simulink model "Arm_2DOF_Step_Input"  (R2021a)
settings: Solver=VariableStepAuto  StartTime=0.0  StopTime=5  MaxStep=0.01  RelTol=1e-3
settings Model: EnablePacing=on  PacingRate=8  Creator=Zicx  LastModifiedBy=Zicx
settings SolverCC: MaxConsecutiveZCs=1500  MaxConsecutiveMinStep=100  ZeroCrossAlgorithm=Adaptive
settings DebuggingCC: SignalInfNanChecking=error  MaskedZcDiagnostic=none  IgnoredZcDiagnostic=none  CheckMatrixSingularityMsg=error  FixptConstUnderflowMsg=warning  FixptConstOverflowMsg=warning  FixptConstPrecisionLossMsg=warning  VectorMatrixConversionMsg=warning  UnderSpecifiedDimensionMsg=error

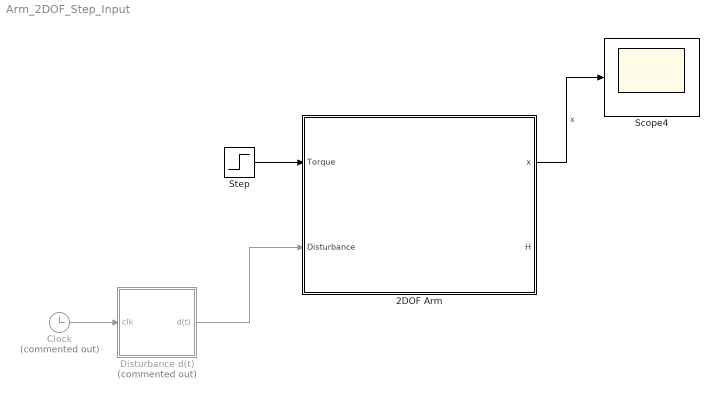
== system Arm_2DOF_Step_Input ==
  2DOF Arm : Subsystem
  Clock : Clock  Commented=on
  Disturbance d(t) : Subsystem  Commented=on
  Scope4 : Scope
  Step : Step  After=[1;1]  SampleTime=0  VectorParams1D=off
  wires:
  Disturbance d(t)/1(d(t)) -> 2DOF Arm/2(Disturbance)
  2DOF Arm/1(x) -> Scope4/1  "x"
  Clock/1 -> Disturbance d(t)/1(clk)
  Step/1 -> 2DOF Arm/1(Torque)

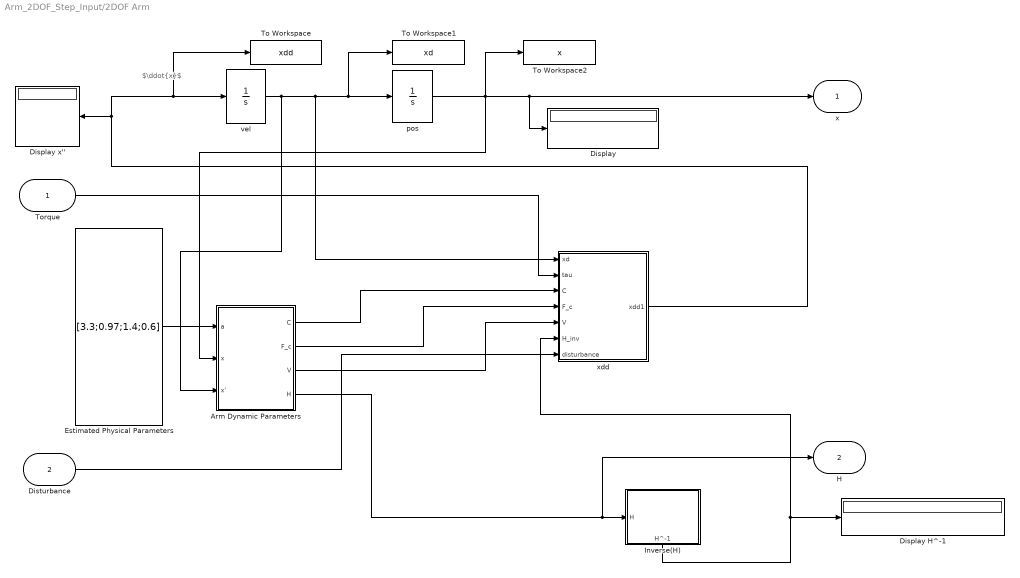
== system Arm_2DOF_Step_Input/2DOF Arm ==
  note: $\ddot{x}$
  Torque : Inport  OutDataTypeStr=double  PortDimensions=[2 1]
  Disturbance : Inport  Port=2  PortDimensions=[2 1]
  Arm Dynamic Parameters : Subsystem
  Display : Display
  Display H^-1 : Display
  Display x'' : Display
  Estimated Physical Parameters : Constant  Value=[3.3;0.97;1.4;0.6]
  Inverse(H) : Subsystem
      settings: PortSchema="{\"entries\":[{\"content\":{\"sides\":[{\"content\":{\"connectorIds\":[\"In1\"]},\"type\":\"ConnectorPlacement.EquallySpacedRectSide\",\"uuid\":\"e93da7b9-99f6-499c-a0cb-6f5b129eec99\"},{\"content\":{\"connectorIds\":[],\"side\":\"RIGHT\"},\"type\":\"ConnectorPlacement.EquallySpacedRectSide\",\"uuid\":\"25c75cce-7d31-4940-9360-78f60f805e3f\"},{\"content\":{\"connectorIds\":[],\"side\":\"TOP\"},\"type\":\"ConnectorPlacement.EquallySpacedRectSide\",\"uuid\":\"446b159b-687d-4bab-aeef-b2e357b1c9d1\"},{\"content\":{\"connectorIds\":[\"Out1\"],\"side\":\"BOTTOM\"},\"type\":\"ConnectorPlacement.EquallySpacedRectSide\",\"uuid\":\"0391da42-abcf-4982-934b-6703b1b91c15\"}]},\"type\":\"ConnectorPlacement.EquallySpacedConnector\",\"uuid\":\"51b5e751-d260-4a7c-9da1-3f7a116869ab\"}],\"packageUris\":[\"http://schema.mathworks.com/mf0/Connector/R2020b\"],\"version\":\"1.0\"}"
  To Workspace : ToWorkspace  VariableName=xdd  SaveFormat=Timeseries  SampleTime=-1
  To Workspace1 : ToWorkspace  VariableName=xd  SaveFormat=Timeseries  SampleTime=-1
  To Workspace2 : ToWorkspace  VariableName=x  SaveFormat=Structure With Time  SampleTime=-1
  pos : Integrator  InitialCondition=[0.3;0.5]  LimitOutput=on  UpperSaturationLimit=2*pi  LowerSaturationLimit=-2 * pi  ContinuousStateAttributes='pos'
  vel : Integrator  LimitOutput=on  UpperSaturationLimit=2*pi  LowerSaturationLimit=-2*pi  ContinuousStateAttributes='vel'
  xdd : Subsystem
  x : Outport  OutDataTypeStr=double  PortDimensions=[2 1]  SampleTime=0
  H : Outport  Port=2
  wires:
  Estimated Physical Parameters/1 -> Arm Dynamic Parameters/1(a)
  Inverse(H)/1(H^-1) -> xdd/6(H_inv), Display H^-1/1
  Arm Dynamic Parameters/4(H) -> H/1, Inverse(H)/1(H)
  vel/1 -> Arm Dynamic Parameters/3(x'), xdd/1(xd), To Workspace1/1, pos/1
  pos/1 -> To Workspace2/1, Arm Dynamic Parameters/2(x), Display/1, x/1
  xdd/1(xdd1) -> Display x''/1, To Workspace/1, vel/1
  Torque/1 -> xdd/2(tau)
  Arm Dynamic Parameters/1(C) -> xdd/3(C)
  Arm Dynamic Parameters/2(F_c) -> xdd/4(F_c)
  Arm Dynamic Parameters/3(V) -> xdd/5(V)
  Disturbance/1 -> xdd/7(disturbance)

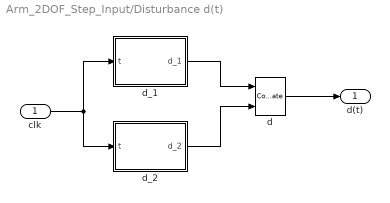
== system Arm_2DOF_Step_Input/Disturbance d(t) ==
  clk : Inport
  d : Concatenate
  d_1 : MATLAB Function  TreatAsAtomicUnit=on
  d_2 : MATLAB Function  TreatAsAtomicUnit=on
  d(t) : Outport
  wires:
  d/1 -> d(t)/1
  clk/1 -> d_2/1(t), d_1/1(t)
  d_1/1(d_1) -> d/1
  d_2/1(d_2) -> d/2

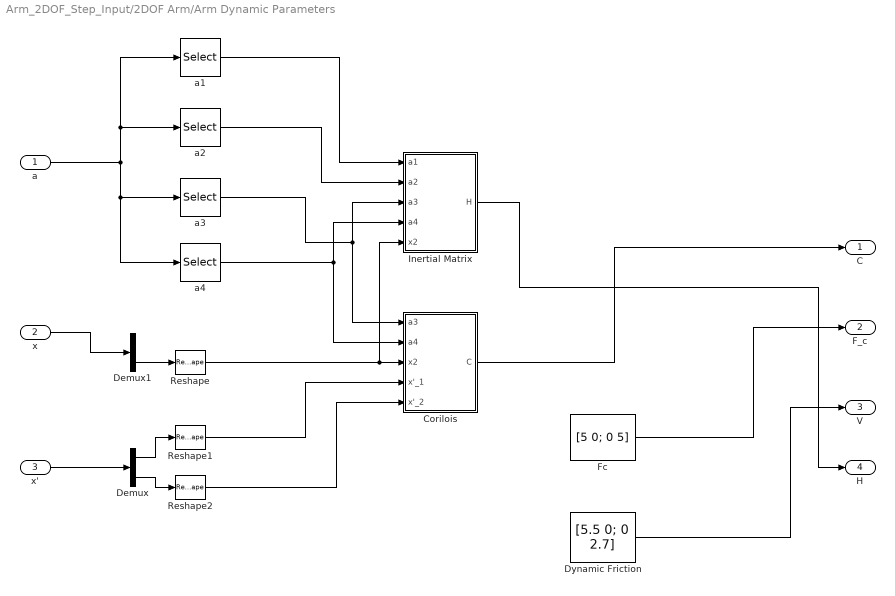
== system Arm_2DOF_Step_Input/2DOF Arm/Arm Dynamic Parameters ==
  a : Inport
  x : Inport  Port=2  PortDimensions=[2 1]
  x' : Inport  Port=3  PortDimensions=[2 1]
  Corilois : Subsystem
  Demux : Demux  Outputs=2
  Demux1 : Demux  Outputs=2
  Dynamic Friction : Constant  Value=[5.5 0; 0 2.7]
  Fc : Constant  Value=[5 0; 0 5]
  Inertial Matrix : Subsystem
  Reshape : Reshape  OutputDimensionality=Customize  OutputDimensions=1
  Reshape1 : Reshape  OutputDimensionality=Customize  OutputDimensions=1
  Reshape2 : Reshape  OutputDimensionality=Customize  OutputDimensions=1
  a1 : Selector  InputPortWidth=4  IndexOptions=Index vector (dialog)  Indices=[1]  OutputSizes=1
  a2 : Selector  InputPortWidth=4  IndexOptions=Index vector (dialog)  Indices=[2]  OutputSizes=1
  a3 : Selector  InputPortWidth=4  IndexOptions=Index vector (dialog)  Indices=[3]  OutputSizes=1
  a4 : Selector  InputPortWidth=4  IndexOptions=Index vector (dialog)  Indices=[4]  OutputSizes=1
  C : Outport
  F_c : Outport  Port=2
  V : Outport  Port=3
  H : Outport  Port=4
  wires:
  a1/1 -> Inertial Matrix/1(a1)
  a/1 -> a1/1, a2/1, a4/1, a3/1
  a3/1 -> Corilois/1(a3), Inertial Matrix/3(a3)
  a4/1 -> Inertial Matrix/4(a4), Corilois/2(a4)
  a2/1 -> Inertial Matrix/2(a2)
  Inertial Matrix/1(H) -> H/1
  Corilois/1(C) -> C/1
  x/1 -> Demux1/1
  Fc/1 -> F_c/1
  Dynamic Friction/1 -> V/1
  x'/1 -> Demux/1
  Demux1/2 -> Reshape/1
  Reshape/1 -> Inertial Matrix/5(x2), Corilois/3(x2)
  Demux/1 -> Reshape1/1
  Demux/2 -> Reshape2/1
  Reshape1/1 -> Corilois/4(x'_1)
  Reshape2/1 -> Corilois/5(x'_2)

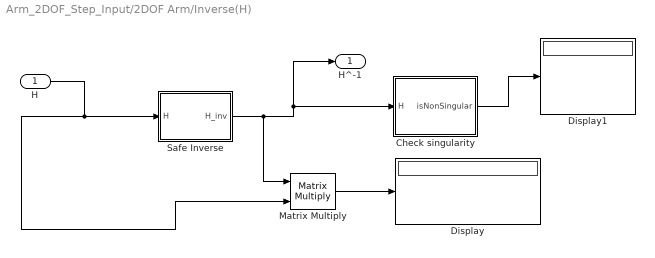
== system Arm_2DOF_Step_Input/2DOF Arm/Inverse(H) ==
  H : Inport  PortDimensions=[2 2]
  Check singularity : MATLAB Function  TreatAsAtomicUnit=on
  Display : Display
  Display1 : Display
  Matrix Multiply : Product  Multiplication=Matrix(*)
  Safe Inverse : MATLAB Function  TreatAsAtomicUnit=on
  H^-1 : Outport
  wires:
  Safe Inverse/1(H_inv) -> Matrix Multiply/1, H^-1/1, Check singularity/1(H)
  H/1 -> Safe Inverse/1(H), Matrix Multiply/2
  Matrix Multiply/1 -> Display/1
  Check singularity/1(isNonSingular) -> Display1/1

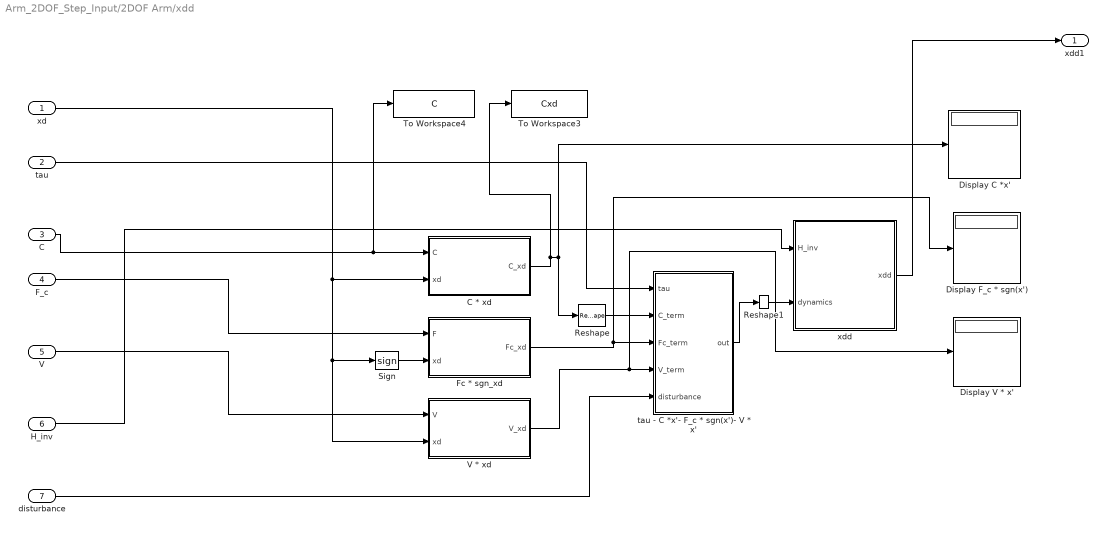
== system Arm_2DOF_Step_Input/2DOF Arm/xdd ==
  xd : Inport
  tau : Inport  Port=2
  C : Inport  Port=3
  F_c : Inport  Port=4
  V : Inport  Port=5
  H_inv : Inport  Port=6
  disturbance : Inport  Port=7
  "C * xd " : MATLAB Function  TreatAsAtomicUnit=on
  Display C *x' : Display
  Display F_c * sgn(x') : Display
  Display V * x' : Display
  Fc * sgn_xd : MATLAB Function  TreatAsAtomicUnit=on
  Reshape : Reshape  OutputDimensionality=Column vector (2-D)
  Reshape1 : Reshape  OutputDimensionality=Column vector (2-D)
  Sign : Signum
  To Workspace3 : ToWorkspace  VariableName=Cxd  SaveFormat=Structure With Time  SampleTime=-1
  To Workspace4 : ToWorkspace  VariableName=C  SaveFormat=Timeseries  SampleTime=-1
  V * xd : MATLAB Function  TreatAsAtomicUnit=on
  "tau - C *x'- F_c * sgn(x')- V * x'  " : MATLAB Function  TreatAsAtomicUnit=on
  xdd : MATLAB Function  TreatAsAtomicUnit=on
  xdd1 : Outport
  wires:
  Sign/1 -> Fc * sgn_xd/2(xd)
  "tau - C *x'- F_c * sgn(x')- V * x'  "/1(out) -> Reshape1/1
  Fc * sgn_xd/1(Fc_xd) -> Display F_c * sgn(x')/1, "tau - C *x'- F_c * sgn(x')- V * x'  "/3(Fc_term)
  xd/1 -> V * xd/2(xd), Sign/1, "C * xd "/2(xd)
  V * xd/1(V_xd) -> Display V * x'/1, "tau - C *x'- F_c * sgn(x')- V * x'  "/4(V_term)
  H_inv/1 -> xdd/1(H_inv)
  Reshape/1 -> "tau - C *x'- F_c * sgn(x')- V * x'  "/2(C_term)
  "C * xd "/1(C_xd) -> To Workspace3/1, Reshape/1, Display C *x'/1
  C/1 -> To Workspace4/1, "C * xd "/1(C)
  Reshape1/1 -> xdd/2(dynamics)
  tau/1 -> "tau - C *x'- F_c * sgn(x')- V * x'  "/1(tau)
  xdd/1(xdd) -> xdd1/1
  disturbance/1 -> "tau - C *x'- F_c * sgn(x')- V * x'  "/5(disturbance)
  V/1 -> V * xd/1(V)
  F_c/1 -> Fc * sgn_xd/1(F)

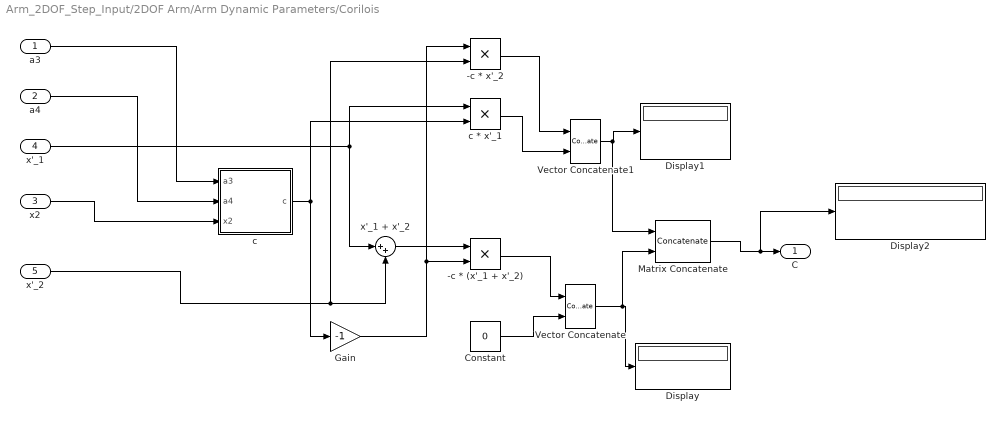
== system Arm_2DOF_Step_Input/2DOF Arm/Arm Dynamic Parameters/Corilois ==
  a3 : Inport
  a4 : Inport  Port=2
  x2 : Inport  Port=3
  x'_1 : Inport  Port=4
  x'_2 : Inport  Port=5
  -c * (x'_1 + x'_2) : Product
  -c * x'_2 : Product
  Constant : Constant  Value=0
  Display : Display
  Display1 : Display
  Display2 : Display
  Gain : Gain  Gain=-1
  Matrix Concatenate : Concatenate  Mode=Multidimensional array  ConcatenateDimension=2
  Vector Concatenate : Concatenate
  Vector Concatenate1 : Concatenate
  c : Subsystem
  c * x'_1 : Product
  x'_1 + x'_2 : Sum  Inputs=|++
  C : Outport
  wires:
  Matrix Concatenate/1 -> Display2/1, C/1
  a4/1 -> c/2(a4)
  a3/1 -> c/1(a3)
  Vector Concatenate1/1 -> Matrix Concatenate/1, Display1/1
  x'_1/1 -> x'_1 + x'_2/1, c * x'_1/1
  x2/1 -> c/3(x2)
  c/1(c) -> Gain/1, c * x'_1/2
  x'_2/1 -> x'_1 + x'_2/2, -c * x'_2/2
  x'_1 + x'_2/1 -> -c * (x'_1 + x'_2)/1
  Vector Concatenate/1 -> Matrix Concatenate/2, Display/1
  Gain/1 -> -c * x'_2/1, -c * (x'_1 + x'_2)/2
  -c * x'_2/1 -> Vector Concatenate1/1
  c * x'_1/1 -> Vector Concatenate1/2
  -c * (x'_1 + x'_2)/1 -> Vector Concatenate/1
  Constant/1 -> Vector Concatenate/2

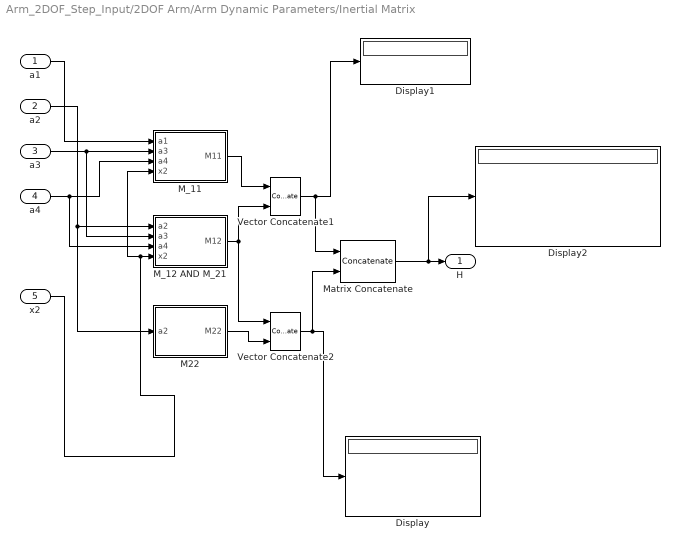
== system Arm_2DOF_Step_Input/2DOF Arm/Arm Dynamic Parameters/Inertial Matrix ==
  a1 : Inport
  a2 : Inport  Port=2
  a3 : Inport  Port=3
  a4 : Inport  Port=4
  x2 : Inport  Port=5
  Display : Display
  Display1 : Display
  Display2 : Display
  M22 : MATLAB Function  TreatAsAtomicUnit=on
  M_11 : MATLAB Function  TreatAsAtomicUnit=on
  M_12 AND M_21 : MATLAB Function  TreatAsAtomicUnit=on
  Matrix Concatenate : Concatenate  Mode=Multidimensional array  ConcatenateDimension=2
  Vector Concatenate1 : Concatenate
  Vector Concatenate2 : Concatenate
  H : Outport
  wires:
  Matrix Concatenate/1 -> Display2/1, H/1
  a1/1 -> M_11/1(a1)
  a3/1 -> M_11/2(a3), M_12 AND M_21/2(a3)
  a4/1 -> M_11/3(a4), M_12 AND M_21/3(a4)
  a2/1 -> M22/1(a2), M_12 AND M_21/1(a2)
  Vector Concatenate2/1 -> Display/1, Matrix Concatenate/2
  M22/1(M22) -> Vector Concatenate2/2
  Vector Concatenate1/1 -> Display1/1, Matrix Concatenate/1
  M_12 AND M_21/1(M12) -> Vector Concatenate2/1, Vector Concatenate1/2
  M_11/1(M11) -> Vector Concatenate1/1
  x2/1 -> M_11/4(x2), M_12 AND M_21/4(x2)

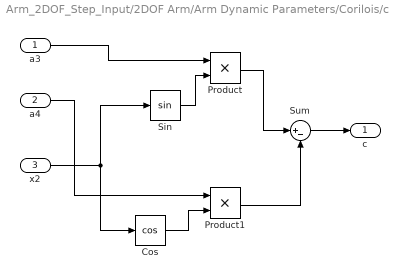
== system Arm_2DOF_Step_Input/2DOF Arm/Arm Dynamic Parameters/Corilois/c ==
  a3 : Inport
  a4 : Inport  Port=2
  x2 : Inport  Port=3
  Cos : Trigonometry  Operator=cos
  Product : Product
  Product1 : Product
  Sin : Trigonometry
  Sum : Sum  Inputs=|+-
  c : Outport
  wires:
  a3/1 -> Product/1
  x2/1 -> Cos/1, Sin/1
  Sin/1 -> Product/2
  a4/1 -> Product1/1
  Cos/1 -> Product1/2
  Product/1 -> Sum/1
  Product1/1 -> Sum/2
  Sum/1 -> c/1

== matlab function Arm_2DOF_Step_Input/2DOF Arm/Inverse(H)/Safe Inverse ==
  data: H input; H_inv output
function H_inv = safe_inverse(H)
    cond_num = cond(H);
    if cond_num > 1e12
        disp('Warning: Matrix is close to singular or badly scaled. Consider using pinv instead.');
        H_inv = pinv(H);
    else
        % Use regularized inverse if necessary
        epsilon = 1e-6; % Small regularization term
        H_reg = H + epsilon * eye(size(H));
        H_inv = inv(H_reg);
        if any(isnan(H_inv), 'all') || any(isinf(H_inv), 'all')
            disp('Warning: Matrix inversion failed. Using pseudoinverse');
            H_inv = pinv(H);
        end
    end
end

== matlab function Arm_2DOF_Step_Input/2DOF Arm/xdd/C * xd  ==
  data: C input; C_xd output; xd input
function C_xd = regulateC_term(C, xd)

    % Define replacement values
    nan_replacement = eps; % A very small positive number
    inf_replacement = realmax; % The largest positive floating-point number
    %negative_inf_replacement = realmin;
    
    % Compute the initial multiplication
    initial_result = C *xd;
    reshape(initial_result, 2, 1);
    
    % Check for NaNs or Infs in the result
    if any(isnan(initial_result)) || any(isinf(initial_result))
        disp("NaN detected in C term!");
    
        % Handle NaNs and Infs in C
        C(isnan(C)) = nan_replacement; % Set NaN elements in C to 0
        C(isinf(C)) = inf_replacement; % Set inf elements in C to 0

        % Handle NaNs and Infs in x_dot
        xd(isnan(xd)) = nan_replacement; % Set NaN elements in x_dot to 0
        xd(isinf(xd)) = inf_replacement; % Set inf elements in x_dot to 0

        % Recompute the multiplication after handling NaNs and Infs
        result = initial_result;
        
        % Ensure the output does not contain NaNs or Infs
        result(isnan(result)) = nan_replacement;
        result(isinf(result)) = inf_replacement;
    else
        % If there are no NaNs or Infs, use the initial result
        result = initial_result;
    end
C_xd = result;
end

== matlab function Arm_2DOF_Step_Input/Disturbance d(t)/d_1 ==
  data: t input; d_1 output
function d_1 = fcn(t)

d_1 = 300* cos(1.7*pi*(t+12)) + 270* sin(pi*t);

== matlab function Arm_2DOF_Step_Input/Disturbance d(t)/d_2 ==
  data: t input; d_2 output
function d_2 = fcn(t)

d_2 = 250 * sin(1.35*pi*(t + 12)) + 300 * cos(2*t);

== matlab function Arm_2DOF_Step_Input/2DOF Arm/Arm Dynamic Parameters/Inertial Matrix/M22 ==
  data: a2 input; M22 output
function M22 = fcn(a2)

M22 = a2;

== matlab function Arm_2DOF_Step_Input/2DOF Arm/Arm Dynamic Parameters/Inertial Matrix/M_11 ==
  data: a1 input; a3 input; a4 input; M11 output; x2 input
function M11 = fcn(a1, a3, a4, x2)
%#codegen

M11 = a1 + 2*a3 * cos(x2)- 2 * a4 * sin(x2);

== matlab function Arm_2DOF_Step_Input/2DOF Arm/Arm Dynamic Parameters/Inertial Matrix/M_12 AND M_21 ==
  data: a2 input; M12 output; a3 input; a4 input; x2 input
function M12 = fcn(a2, a3, a4, x2)

M12 = a2 + a3 * cos(x2) + a4 * sin(x2);

== matlab function Arm_2DOF_Step_Input/2DOF Arm/xdd/xdd ==
  data: H_inv input; xdd output; dynamics input
function xdd = xdd(H_inv, dynamics)

    % Define replacement values
    nan_replacement = eps; % A very small positive number
    inf_replacement = realmax; % The largest positive floating-point number
    
    % Compute the initial multiplication
    initial_xdd = H_inv * dynamics;
    
    % Check for NaNs or Infs in the result
    if any(isnan(initial_xdd)) || any(isinf(initial_xdd))
        disp("NaN detected!");
        disp(H_inv);
        disp(dynamics);
        disp(initial_xdd);
    
        % Handle NaNs and Infs in H_inv
        H_inv(isnan(H_inv)) = nan_replacement; % Set NaN elements in H_inv to 0
        H_inv(isinf(H_inv)) = inf_replacement; % Set inf elements in H_inv to 0

        % Handle NaNs and Infs in dynamics
        dynamics(isnan(dynamics)) = nan_replacement; % Set NaN elements in dynamics to 0
        dynamics(isinf(dynamics)) = inf_replacement; % Set inf elements in dynamics to 0

        % Recompute the multiplication after handling NaNs and Infs
        result = H_inv * dynamics;
        
        % Ensure the output does not contain NaNs or Infs
        result(isnan(result)) = nan_replacement;
        result(isinf(result)) = inf_replacement;
    else
        % If there are no NaNs or Infs, use the initial result
        result = initial_xdd;
    end
xdd = reshape(result, 2, 1);
end

== matlab function Arm_2DOF_Step_Input/2DOF Arm/Inverse(H)/Check singularity ==
  data: H input; isNonSingular output
function isNonSingular = checkNonSingular(H)
    % H is the input matrix
    determinant = det(H);
    if determinant ~= 0
        isNonSingular = 1;
    else
        isNonSingular = 0;
    end
end

== matlab function Arm_2DOF_Step_Input/2DOF Arm/xdd/tau - C *x'- F_c * sgn(x')- V * x'   ==
  data: tau input; out output; C_term input; Fc_term input; V_term input; disturbance input
function out = dynamics(tau, C_term, Fc_term, V_term, disturbance)
    % Define replacement values
    nan_replacement = eps; % A very small positive number
    inf_replacement = realmax; % The largest positive floating-point number
    
    % Compute result
    result = tau - C_term - Fc_term - V_term - disturbance;
    
    % Ensure the output does not contain NaNs or Infs
    result(isnan(result)) = nan_replacement;
    result(isinf(result)) = inf_replacement;

    out = result;
    out = reshape(out, 2, 1);
end

== matlab function Arm_2DOF_Step_Input/2DOF Arm/xdd/Fc * sgn_xd ==
  data: F input; Fc_xd output; xd input
function Fc_xd = regulateFc_xd(F, xd)

    % Define replacement values
    nan_replacement = eps; % A very small positive number
    inf_replacement = realmax; % The largest positive floating-point number
    
    % Compute the initial multiplication
    initial_result = F *xd;
    reshape(initial_result, 2, 1);
    
    % Check for NaNs or Infs in the result
    if any(isnan(initial_result)) || any(isinf(initial_result))
        disp("NaN detected in F term!");
    
        % Handle NaNs and Infs in C
        F(isnan(F)) = nan_replacement; % Set NaN elements in C to 0
        F(isinf(F)) = inf_replacement; % Set inf elements in C to 0

        % Handle NaNs and Infs in x_dot
        xd(isnan(xd)) = nan_replacement; % Set NaN elements in x_dot to 0
        xd(isinf(xd)) = inf_replacement; % Set inf elements in x_dot to 0

        % Recompute the multiplication after handling NaNs and Infs
        result = initial_result;
        
        % Ensure the output does not contain NaNs or Infs
        result(isnan(result)) = nan_replacement;
        result(isinf(result)) = inf_replacement;
    else
        % If there are no NaNs or Infs, use the initial result
        result = initial_result;
    end
Fc_xd = result;
end

== matlab function Arm_2DOF_Step_Input/2DOF Arm/xdd/V * xd ==
  data: V input; V_xd output; xd input
function V_xd = regulateV_xd(V, xd)

    % Define replacement values
    nan_replacement = eps; % A very small positive number
    inf_replacement = realmax; % The largest positive floating-point number
    
    % Compute the initial multiplication
    initial_result = V *xd;
    reshape(initial_result, 2, 1);
    
    % Check for NaNs or Infs in the result
    if any(isnan(initial_result)) || any(isinf(initial_result))
        disp("NaN detected in V term!");
    
        % Handle NaNs and Infs in C
        V(isnan(V)) = nan_replacement; % Set NaN elements in C to 0
        V(isinf(V)) = inf_replacement; % Set inf elements in C to 0

        % Handle NaNs and Infs in x_dot
        xd(isnan(xd)) = nan_replacement; % Set NaN elements in x_dot to 0
        xd(isinf(xd)) = inf_replacement; % Set inf elements in x_dot to 0

        % Recompute the multiplication after handling NaNs and Infs
        result = initial_result;
        
        % Ensure the output does not contain NaNs or Infs
        result(isnan(result)) = nan_replacement;
        result(isinf(result)) = inf_replacement;
    else
        % If there are no NaNs or Infs, use the initial result
        result = initial_result;
    end
V_xd = result;
end
